simulink model "my_dm6437evmsurveil_tcpip"  (Simulink 7.1)
settings: Solver=FixedStepDiscrete  SolverMode=SingleTasking  StartTime=0.0  StopTime=inf  RelTol=1e-3
PostLoadFcn:
  | c6000demoscallback
libraries: etargetslib x2, c6000demolib x1, dspbioslib x1
CloseFcn:
  | clear vR3 vG3 vB3
settings Model: Creator=don  LastModifiedBy=karin
settings SolverCC: PositivePriorityOrder=on
settings DataIOCC: LimitDataPoints=off  SaveOutput=off  SaveTime=off  SignalLoggingName=sigsOut
settings OptimizationCC: EnforceIntegerDowncast=off  LocalBlockOutputs=off  OptimizeModelRefInitCode=on  BufferReusableBoundary=off
settings DebuggingCC: CheckExecutionContextPreStartOutputMsg=on  CheckExecutionContextRuntimeOutputMsg=on  SignalResolutionControl=TryResolveAllWithWarning  SolverPrmCheckMsg=none  MultiTaskDSMMsg=warning  MultiTaskCondExecSysMsg=none  SigSpecEnsureSampleTimeMsg=none
settings HardwareCC: ProdBitPerLong=40  ProdIntDivRoundTo=Zero  ProdEndianess=LittleEndian  ProdHWDeviceType=TI C6000  TargetHWDeviceType=32-bit Generic
settings ModelReferenceCC: UpdateModelReferenceTargets=IfOutOfDate
settings RTWCC: SystemTargetFile=ccslink_ert.tlc  GenerateMakefile=off  TemplateMakefile=ccslink_ert.tmf  Description=Embedded IDE Link CC (ERT) code generation for TMS320(TM) DSP platforms  ProcessScript=ccslink_ert_make_rtw_hook  IncludeERTFirstTime=on
settings CodeAppCC: IgnoreCustomStorageClasses=off
settings ERTTgtLinkCCS: TargetFcnLib=ansi_tfl_tmw_new.mat  TargetFunctionLibrary=ANSI_C  UtilityFuncGeneration=Auto  GenerateFullHeader=on  GenerateSampleERTMain=off  GenerateTestInterfaces=off  IsPILTarget=off  ModelReferenceCompliant=on  CompOptLevelCompliant=off  IncludeMdlTerminateFcn=on  CombineOutputUpdateFcns=on  SuppressErrorStatus=off  IncludeFileDelimiter=Auto  ERTCustomFileBanners=on  SupportAbsoluteTime=on  LogVarNameModifier=rt_  MatFileLogging=off  MultiInstanceERTCode=off  SupportNonFinite=on  SupportComplex=on  PurelyIntegerCode=off  SupportContinuousTime=off  SupportNonInlinedSFcns=off  EnableShiftOperators=on  ParenthesesLevel=Nominal  PortableWordSizes=off  ModelStepFunctionPrototypeControlCompliant=off  AutosarCompliant=off  GenerateErtSFunction=off  GenerateASAP2=off  ExtMode=off  ExtModeTransport=0  ExtModeStaticAlloc=on  ExtModeStaticAllocSize=1000000  ExtModeTesting=off  ExtModeMexFile=ext_comm  ExtModeIntrfLevel=Level1  InlinedParameterPlacement=NonHierarchical  TargetOS=BareBoardExample  MultiInstanceErrorCode=Error  RateGroupingCode=on  RootIOFormat=Individual arguments  RTWCAPISignals=off  RTWCAPIParams=off  RTWCAPIStates=off  ERTSrcFileBannerTemplate=ert_code_template.cgt  ERTHdrFileBannerTemplate=ert_code_template.cgt  ERTDataSrcFileTemplate=ert_code_template.cgt  ERTDataHdrFileTemplate=ert_code_template.cgt  ERTCustomFileTemplate=example_file_process.tlc  ModuleNamingRule=Unspecified  SignalDisplayLevel=10  ParamTuneLevel=10  GlobalDataDefinition=Auto  DataDefinitionFile=global.c  GlobalDataReference=Auto  DataReferenceFile=global.h  GRTInterface=off  PreserveExpressionOrder=off  PreserveIfCondition=off  EnableUserReplacementTypes=off  MemSecPackage=--- None ---  MemSecDataConstants=Default  MemSecDataIO=Default  MemSecDataInternal=Default  MemSecDataParameters=Default  MemSecFuncInitTerm=Default  MemSecFuncExecute=Default  exportIDEObj=on  ideObjName=CCS_Obj  oldideObjName=CCS_Obj  ideObjTimeout=10  oldideObjTimeout=10  ideObjBuildTimeout=1000  oldideObjBuildTimeout=1000  ProfileGenCode=off  ProfileNumSamples=100  InlineDSPBlks=on  projectOptions=Custom  debugCompilerOptions="-g -d\"_DEBUG\""  releaseCompilerOptions=-o2  customCompilerOptions=-o2 --mem_model:data=far  compilerOptionsStr=-o2 --mem_model:data=far  getCompilerOptions=off  getLinkerOptions=off  systemStackSize=8192  buildAction=Build  overrunNotificationMethod=None  overrunNotificationFcn=myfunction  oldoverrunNotificationFcn=myfunction  configurePIL=off  configPILBlockAction=None

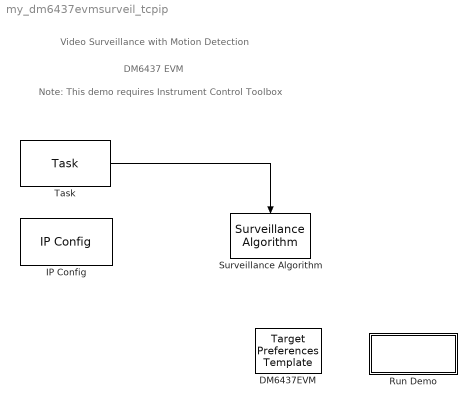
== system my_dm6437evmsurveil_tcpip ==
  note: Video Surveillance with Motion Detection
  note: DM6437 EVM
  note: Note: This demo requires Instrument Control Toolbox
  DM6437EVM : etargetslib/Target Preferences Template  Tag=ccslinktgtpref  SystemSampleTime=-1
  IP Config : etargetslib/IP Config  boardType=DM6437EVM  daughterCard=Internal EMAC  tcpipStackDir=$(NDK_INSTALL_DIR)\packages\ti\ndk  enetIntNum=13  memSegment=DDR  enablePrintfs=on  dhcpEnabled=on  IPAddr=100.100.100.2  subnetMask=255.255.255.0  gatewayIP=100.100.100.1  dnsServerIP=0.0.0.0  domainName=mathworks.net  hostName=dm6437evm
  Run Demo : Subsystem  Description=Controls host-side RTDX processing.  AncestorBlock=demo_controls/Run Demo
      settings: OpenFcn=my_tcpip_surveil_script('my_pc_surveil_tcpip');
      mask Display: disp(sprintf('Build / Reload\n& Run'))
  Surveillance Algorithm : c6000demolib/Surveillance Algorithm  SystemSampleTime=-1
  Task : dspbioslib/Task  SystemSampleTime=-1  taskName=Task0  taskPriority=1  taskExecutionOrder=1  taskStackSize=8192  stackMemSegment=IRAM  monitorStackUse=off  taskYield=off  parentmanaget=on  tickres=1/1000  ticklen=32bits  taskTrigger=off
  wires:
  Task/1 -> Surveillance Algorithm/Trigger

== system my_dm6437evmsurveil_tcpip/Run Demo ==
